simulink model "Controller_bis (1)"  (R2019b)
settings: Solver=ode4  StartTime=0.0  StopTime=10  FixedStep=0.01  RelTol=1e-3  EnableMultiTasking=on
values from neighbouring files (symbols this model uses):
  m = 0.5    [LCS_freq.m]    (also in LoopShaping_TP.m = 2)
libraries: simulink x1
settings Model: Creator=Thomas  LastModifiedBy=Ivan
settings DataIOCC: LimitDataPoints=on  SaveFormat=Array  ReturnWorkspaceOutputs=off
settings OptimizationCC: LifeSpan=inf
settings DebuggingCC: SolverPrmCheckMsg=warning  SFUnexpectedBacktrackingDiag=warning  SFNoUnconditionalDefaultTransitionDiag=warning  SFExecutionAtInitializationDiag=none  ArithmeticOperatorsInVariantConditions=warning
settings HardwareCC: ProdBitPerPointer=32  ProdBitPerSizeT=32  ProdBitPerPtrDiffT=32  ProdLargestAtomicFloat=None  ProdIntDivRoundTo=Undefined  ProdEndianess=Unspecified  ProdWordSize=32  ProdHWDeviceType=32-bit Generic
settings ModelReferenceCC: PropagateSignalLabelsOutOfModel=off
settings SFSimCC: SimUseLocalCustomCode=off  CustomCodeUndefinedFunction=UseInterfaceOnly
settings RTWCC: RTWUseLocalCustomCode=off
settings CodeAppCC: StateflowObjectComments=on
settings GRTTargetCC: TargetLangStandard=C89/C90 (ANSI)
settings ConfigComp: CovMetricSettings=dw  CovSaveCumulativeToWorkspaceVar=on  CovSaveSingleToWorkspaceVar=on  CovExternalEMLEnable=off  CovSFcnEnable=off

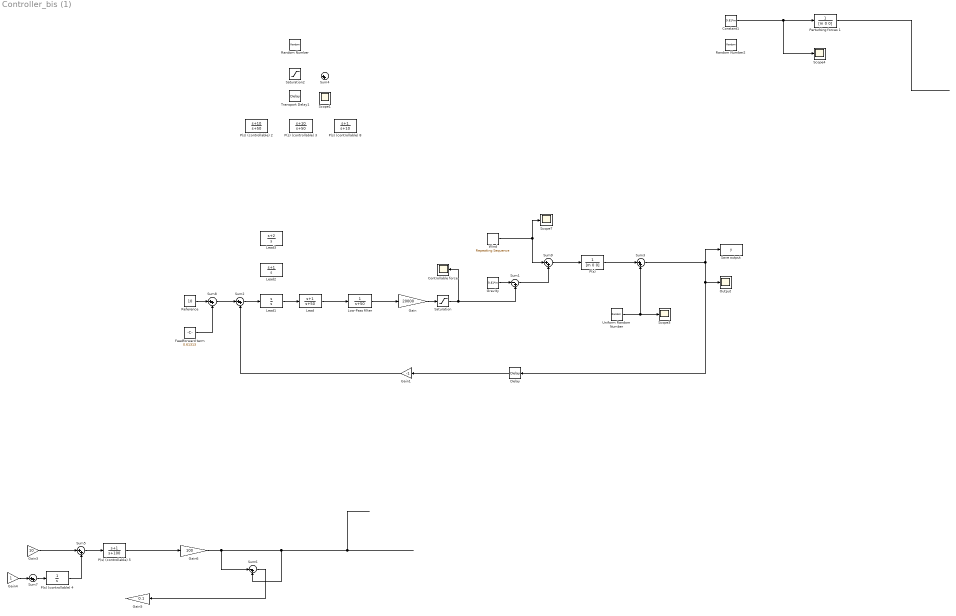
== system Controller_bis (1) ==
  Constant1 : Constant  Value=9.81*m
  Controllable force : Scope
  Delay : TransportDelay  DelayTime=0.02
  Feedforward term : Constant  Value=0.61313
  Gain : Gain  Gain=20000
  Gain1 : Gain  Gain=-1
  Gain3 : Gain  Gain=10
  Gain4 : Gain
  Gain5 : Gain  Gain=0.1
  Gain6 : Gain  Gain=100
  Gravity : Constant  Value=9.81*m
  Lead : TransferFcn  Numerator=[1 1]  Denominator=[1 50]
  Lead1 : TransferFcn  Numerator=[1 0]  Denominator=[1 0]
  Lead2 : TransferFcn  Numerator=[1 1]  Denominator=[1 0]
  Lead3 : TransferFcn  Numerator=[1 2]  Denominator=[1 0]
  Low-Pass filter : TransferFcn  Denominator=[1 50]
  Output : Scope
  "P(s) " : TransferFcn  Denominator=[m 0 0]
  P(s) (controllable) 2 : TransferFcn  Numerator=[1 10]  Denominator=[1 50]
  P(s) (controllable) 3 : TransferFcn  Numerator=[1 10]  Denominator=[1 50]
  P(s) (controllable) 4 : TransferFcn  Denominator=[1 0]
  P(s) (controllable) 5 : TransferFcn  Numerator=[1 1]  Denominator=[1 100]
  P(s) (controllable) 8 : TransferFcn  Numerator=[1 1]  Denominator=[1 10]
  Perturbing forces 1 : TransferFcn  Denominator=[m 0 0]
  Random Number : RandomNumber  Seed=3  SampleTime=0.01
  Random Number2 : RandomNumber  Seed=3  SampleTime=0.01
  "Reference " : Constant  Value=10
  Saturation : Saturate  UpperLimit=10  LowerLimit=-10
  Saturation2 : Saturate
  Save output : ToWorkspace  VariableName=y  SaveFormat=Timeseries  SampleTime=-1
  Scope{1,3..4,7} (4 alike) : Scope
  Sum1 : Sum  Inputs=|-+
  Sum{2..5,7..9} (7 alike) : Sum  Inputs=|++
  Sum6 : Sum  Inputs=|-+
  Transport Delay1 : TransportDelay
  Uniform Random Number : UniformRandomNumber  Minimum=-0.05  Maximum=0.05  SampleTime=0.01
  Wind : simulink/Sources/Repeating Sequence  rep_seq_t=[0 2]  rep_seq_y=[0 2]
  wires:
  Gain1/1 -> Sum2/2
  ? -> Gain4/1, Gain3/1
  Sum5/1 -> P(s) (controllable) 5/1
  P(s) (controllable) 4/1 -> Sum5/2
  Sum6/1 -> Gain5/1
  P(s) (controllable) 5/1 -> Gain6/1
  Gain4/1 -> Sum7/1
  Sum7/1 -> P(s) (controllable) 4/1
  Gain3/1 -> Sum5/1
  Gain6/1 -> Sum6/2, Sum6/1
  Gain/1 -> Saturation/1
  Lead/1 -> Low-Pass filter/1
  Low-Pass filter/1 -> Gain/1
  Sum3/1 -> Delay/1, Output/1, Save output/1
  Constant1/1 -> Scope4/1, Perturbing forces 1/1
  Perturbing forces 1/1 -> ?
  Saturation/1 -> Sum1/2, Controllable force/1
  Uniform Random Number/1 -> Sum3/2, Scope3/1
  "P(s) "/1 -> Sum3/1
  Sum8/1 -> Sum2/1
  "Reference "/1 -> Sum8/1
  Sum1/1 -> Sum9/2
  Sum9/1 -> "P(s) "/1
  Wind/1 -> Sum9/1, Scope7/1
  Gravity/1 -> Sum1/1
  Feedforward term/1 -> Sum8/2
  Delay/1 -> Gain1/1
  Sum2/1 -> Lead1/1
  Lead1/1 -> Lead/1
